simulink model "L4_SIM"  (R2018a)
settings: Solver=ode1  StartTime=0.0  StopTime=60  FixedStep=GLB_FIXED_STEP_SIZE_CPV  RelTol=1e-3  EnableMultiTasking=on
undefined symbols (not defined in the file or in its folder): Cf, Chassis, Cr, CYCLE_ACC1_2A__AdaptiveCruiseCtrlMode, CYCLE_ACC1_2A__AdaptiveCruiseCtrlSetSpeed, CYCLE_CCVS1_00__CruiseCtrlSetSpeed, CYCLE_CCVS1_00__WheelBasedVehicleSpeed, CYCLE_EEC1_00__EngSpeed, CYCLE_ETC1_00__TransDrivelineEngaged, CYCLE_ETC2_00__TransActualGearRatio, CYCLE_ETC7_03__TransMode1Indicator, CYCLE_GPS_Latitude, CYCLE_GPS_Longitude, CYCLE_LFE1_00__EngFuelRate, CYCLE_Net_Engine_Percent_Torque, CYCLE_SSI2_03__PitchAngleExRange, CYCLE_TIME, CYCLE_UTM_Origin_X, CYCLE_UTM_Origin_Y, CYCLE_Vehicle_Distance, DiscIntNeverNeededParam, ENUM_J1939_PCC_STATE_T, ENUM_J1939_SWITCH_T, ENUM_STEERING_WHEEL_ANGLE_SENSOR_TYPE_T, GLB_FIXED_STEP_SIZE_CPV, GLB_TRANS_LOSS_TRQ_GEAR_STEP_MPV, GLB_TRANS_LOSS_TRQ_SPD_STEP_MPV, GLB_TRANS_LOSS_TRQ_TABLE_DATA_MPV, GLB_TRANS_LOSS_TRQ_TRQ_STEP_MPV, GLB_VEHICLE_CONFIG_ACCEL_PED_GATEWAY_APV, heading_0, Iz, L4_Controller, lf, lr, position_0, ptc_matlab_lib, STEERCTRL_10ms, SUB_ECU_L4_MABX, SUB_L4_Task_10ms, SUB_L4_Task_10ms_SUB_STEERCTRL, SUB_PLANT_Chassis, Task_10ms, Vx_0
libraries: EmE_MBD_Blockset x81, PTC_MBDS_LIB x71, simulink x38, simulink_extras x1, SUB_L4_Task_10000ms x1, SUB_L4_Task_1000ms x1, SUB_L4_Task_100ms x1, SUB_L4_Task_10ms_SUB_APTC x1, SUB_L4_Task_10ms_SUB_BRKPEDARB x1, SUB_L4_Task_10ms_SUB_FAULT_MANAGER x1, SUB_L4_Task_10ms_SUB_STATE_CONTROL x1, simulink_need_slupdate x1
(part 6 of 6)

== system L4_SIM/Controllers/Virtual_Controllers/L4_MABX/L4_Controller/Task_10ms/Vehicle_speed_target/Determine_sigmoid_vehicle_speed_profile/Select_vehicle_speed_target_value ==
  Vehicle_speed_initial : Inport
  F_Enable : Inport  Port=2
  Distance_m : Inport  Port=3
  Vehicle_speed : Inport  Port=4
  Vehicle_speed_target : Inport  Port=5
  Position_vector_m : Inport  Port=6
  Vehicle_speed_vector_kph : Inport  Port=7
  MIN_VSPD_SIGMOID_INITIAL_KPH_APV : Inport  Port=8
  MIN_VSPD_SIGMOID_FINAL_KPH_APV : Inport  Port=9
  CPV1 : EmE_MBD_Blockset/Sources/CPV  conval=0.1
      settings: SourceProductName=PACCAR EmE MBD Blockset
  Gain1 : Gain  Gain=1/3.6
  If_Then_Else : EmE_MBD_Blockset/Signal Routing/If_Then_Else
      settings: SourceProductName=PACCAR EmE MBD Blockset
  Integrators : Subsystem
  Logical Operator : EmE_MBD_Blockset/Logic and Bit Operations/Logical Operator  Operator=OR  Inputs=2
      settings: SourceProductName=PACCAR EmE MBD Blockset
  Logical Operator2 : EmE_MBD_Blockset/Logic and Bit Operations/Logical Operator  Operator=AND  Inputs=2
      settings: SourceProductName=PACCAR EmE MBD Blockset
  Lookup Table Dynamic : simulink/Lookup Tables/Lookup Table Dynamic  LookUpMeth=Interpolation-Use End Values  OutDataType=fixdt('double')  OutScaling=[]  OutputDataTypeScalingMode=Specify via dialog  OutDataTypeStr=double  DoSatur=off
      settings: SourceProductName=Simulink
  Relational Operator : EmE_MBD_Blockset/Logic and Bit Operations/Relational Operator  func===
      settings: SourceProductName=PACCAR EmE MBD Blockset
  Relational Operator1 : EmE_MBD_Blockset/Logic and Bit Operations/Relational Operator  func=<
      settings: SourceProductName=PACCAR EmE MBD Blockset
  Relational Operator2 : EmE_MBD_Blockset/Logic and Bit Operations/Relational Operator  func=<
      settings: SourceProductName=PACCAR EmE MBD Blockset
  Relational Operator3 : EmE_MBD_Blockset/Logic and Bit Operations/Relational Operator  func=<
      settings: SourceProductName=PACCAR EmE MBD Blockset
  Terminator : Terminator
  Vehicle_speed_profile_sigmoid : Outport
  wires:
  Logical Operator2/1 -> Integrators/3(F_SetMax)  "F_set_max_distance_accumulated"
  CPV1/1 -> Relational Operator3/2
  Relational Operator1/1 -> Logical Operator/2
  Logical Operator/1 -> Logical Operator2/1
  Relational Operator3/1 -> Logical Operator/1
  Relational Operator/1 -> If_Then_Else/1
  Gain1/1 -> Integrators/2(Vehicle_speed_ms)
  Integrators/2(Distance_accumulated_m) -> Relational Operator/1, Lookup Table Dynamic/1
  MIN_VSPD_SIGMOID_FINAL_KPH_APV/1 -> Relational Operator2/2
  MIN_VSPD_SIGMOID_INITIAL_KPH_APV/1 -> Relational Operator1/2
  Relational Operator2/1 -> Logical Operator2/2
  Vehicle_speed_initial/1 -> Relational Operator1/1
  F_Enable/1 -> Integrators/1(F_Reset)
  Lookup Table Dynamic/1 -> If_Then_Else/3
  Vehicle_speed_vector_kph/1 -> Lookup Table Dynamic/3
  Integrators/1(Elasped_time_secs) -> Terminator/1
  Position_vector_m/1 -> Lookup Table Dynamic/2
  Vehicle_speed/1 -> Gain1/1, Relational Operator3/1
  Distance_m/1 -> Integrators/4(Max), Relational Operator/2
  If_Then_Else/1 -> Vehicle_speed_profile_sigmoid/1  "Vehicle_speed_profile_sigmoid"
  Vehicle_speed_target/1 -> Relational Operator2/1, If_Then_Else/2

== system L4_SIM/Plant/PlantModel/Chassis/Chassis_SL/Chassis/Vehicle Dynamics/Aero/Signed square ==
  In1 : Inport
  Math Function : Math  Operator=square  SaturateOnIntegerOverflow=on
  Product : Product  RndMeth=Zero
  Sign : Signum  ZeroCross=off
  Out1 : Outport
  wires:
  Product/1 -> Out1/1
  Sign/1 -> Product/2
  Math Function/1 -> Product/1
  In1/1 -> Sign/1, Math Function/1

== system L4_SIM/Controllers/Virtual_Controllers/L4_MABX/L4_Controller/Task_10ms/STEERCTRL_10ms/PID/PID/PID ==
  Init : Inport
  Reset_Integral : Inport  Port=2
  Err : Inport  Port=3
  K : Inport  Port=4
  Ti : Inport  Port=5
  Td : Inport  Port=6
  Ts : Inport  Port=7
  Sat_state : Inport  Port=8
  Add : Sum
  Add1 : Sum  Inputs=+++
  Add3 : Sum  Inputs=+-
  AntiWindup : Subsystem
  Divide : Product  Inputs=*/
  Divide1 : Product  Inputs=**/
  Product : Product  RndMeth=Zero
  Product1 : Product  RndMeth=Zero
  Switch : Switch  Criteria=u2 ~= 0
  Unit Delay : UnitDelay  SampleTime=-1
  Unit Delay1 : UnitDelay  SampleTime=-1
  Out1 : Outport
  P_Out : Outport  Port=2
  I_Out : Outport  Port=3
  D_Out1 : Outport  Port=4
  wires:
  Add3/1 -> D_Out1/1, Add1/3
  Unit Delay1/1 -> Add3/2
  Divide1/1 -> Unit Delay1/1, Add3/1
  [KpError] -> Divide1/2
  Td/1 -> Divide1/1
  Add1/1 -> Out1/1
  Add/1 -> I_Out/1, Add1/2, Switch/3
  Switch/1 -> Unit Delay/1
  Unit Delay/1 -> Add/2
  Divide/1 -> Product1/2
  Ti/1 -> Divide/2
  Ts/1 -> Divide/1, Divide1/3
  Product/1 -> [KpError], P_Out/1, Add1/1, Product1/1
  K/1 -> Product/2
  Err/1 -> Product/1
  Init/1 -> Switch/1
  Reset_Integral/1 -> Switch/2
  AntiWindup/1(I_update_clp) -> Add/1
  Product1/1 -> AntiWindup/1(I_update)
  Sat_state/1 -> AntiWindup/2(Sat_state)

== system L4_SIM/Controllers/Virtual_Controllers/L4_MABX/L4_Controller/Task_10ms/Vehicle_speed_target/Determine_sigmoid_vehicle_speed_profile/Determine_inhibit_sigmoid_vehicle_speed_profile/Capture_initial_vehicle_speed_value ==
  Vehicle_speed : Inport
  F_Enable : Inport  Port=2
  If_Then_Else : EmE_MBD_Blockset/Signal Routing/If_Then_Else
      settings: SourceProductName=PACCAR EmE MBD Blockset
  Unit_Delay : UnitDelay  SampleTime=-1
      settings: AttributesFormatString=IC: %<vinit>
  Vehicle_speed_initial : Outport
  wires:
  Vehicle_speed/1 -> If_Then_Else/2
  Unit_Delay/1 -> If_Then_Else/3
  F_Enable/1 -> If_Then_Else/1
  If_Then_Else/1 -> Vehicle_speed_initial/1, Unit_Delay/1  "Vehicle_speed_initial"

== system L4_SIM/Controllers/Virtual_Controllers/L4_MABX/L4_Controller/Task_10ms/Vehicle_speed_target/Determine_sigmoid_vehicle_speed_profile/Select_vehicle_speed_target_value/Integrators ==
  F_Reset : Inport
  Vehicle_speed_ms : Inport  Port=2
  F_SetMax : Inport  Port=3
  Max : Inport  Port=4
  CPV : EmE_MBD_Blockset/Sources/CPV  conval=1
      settings: SourceProductName=PACCAR EmE MBD Blockset
  CPV1 : EmE_MBD_Blockset/Sources/CPV  conval=1
      settings: SourceProductName=PACCAR EmE MBD Blockset
  CPV2 : EmE_MBD_Blockset/Sources/CPV  conval=1
      settings: SourceProductName=PACCAR EmE MBD Blockset
  CalculateDistance : Subsystem
  Discrete-Time Integrator : EmE_MBD_Blockset/Discrete/Discrete-Time Integrator  integrator_method_sel=Backward Euler
      settings: AttributesFormatString=%<integrator_method_sel>  SourceProductName=PACCAR EmE MBD Blockset
  dT : EmE_MBD_Blockset/Sources/dT
      settings: SourceProductName=PACCAR EmE MBD Blockset
  dT1 : EmE_MBD_Blockset/Sources/dT
      settings: SourceProductName=PACCAR EmE MBD Blockset
  Elasped_time_secs : Outport
  Distance_accumulated_m : Outport  Port=2
  wires:
  F_SetMax/1 -> CalculateDistance/5(F_SetMax)
  Max/1 -> CalculateDistance/6(Max)
  CPV2/1 -> Discrete-Time Integrator/2
  CPV1/1 -> CalculateDistance/3(K)
  dT1/1 -> CalculateDistance/4(dT)
  Discrete-Time Integrator/1 -> Elasped_time_secs/1  "Elasped_time_secs"
  F_Reset/1 -> Discrete-Time Integrator/1, CalculateDistance/1(F_Reset)
  Vehicle_speed_ms/1 -> CalculateDistance/2(U)
  CPV/1 -> Discrete-Time Integrator/3
  CalculateDistance/1(Y) -> Distance_accumulated_m/1  "Distance_accumulated_m"
  dT/1 -> Discrete-Time Integrator/4

== system L4_SIM/Controllers/Virtual_Controllers/L4_MABX/L4_Controller/Task_10ms/STEERCTRL_10ms/PID/PID/PID/AntiWindup ==
  I_update : Inport
  Sat_state : Inport  Port=2
  Constant : Constant  Value=0
  Constant1 : Constant
  Constant2 : Constant  Value=-1
  Constant3 : Constant
  Constant4 : Constant  Value=-1
  Constant5 : Constant  Value=2
  Logical Operator : Logic  Operator=OR  AllPortsSameDT=off  OutDataTypeStr=boolean
  Logical Operator1 : Logic  AllPortsSameDT=off  OutDataTypeStr=boolean
  Logical Operator2 : Logic  AllPortsSameDT=off  OutDataTypeStr=boolean
  Logical Operator3 : Logic  AllPortsSameDT=off  OutDataTypeStr=boolean
  Relational Operator1 : RelationalOperator  Operator=~=  OutDataTypeStr=boolean  RndMeth=Nearest
  Relational Operator2 : RelationalOperator  Operator=~=  OutDataTypeStr=boolean  RndMeth=Nearest
  Relational Operator3 : RelationalOperator  Operator===  OutDataTypeStr=boolean  RndMeth=Nearest
  Relational Operator4 : RelationalOperator  Operator===  OutDataTypeStr=boolean  RndMeth=Nearest
  Relational Operator5 : RelationalOperator  Operator=~=  OutDataTypeStr=boolean  RndMeth=Nearest
  Sign1 : Signum
  Switch1 : Switch  Criteria=u2 ~= 0
  I_update_clp : Outport
  wires:
  Switch1/1 -> I_update_clp/1
  I_update/1 -> Sign1/1, Switch1/1
  Constant1/1 -> Relational Operator1/2
  Sat_state/1 -> Relational Operator1/1, Relational Operator2/1, [Sat_state]
  Constant2/1 -> Relational Operator2/2
  Sign1/1 -> Relational Operator4/2, Relational Operator3/2
  Constant3/1 -> Relational Operator3/1
  Constant4/1 -> Relational Operator4/1
  Relational Operator2/1 -> Logical Operator1/2
  Relational Operator4/1 -> Logical Operator1/1
  Relational Operator3/1 -> Logical Operator2/2
  Relational Operator1/1 -> Logical Operator2/1
  Logical Operator1/1 -> Logical Operator/1
  Logical Operator2/1 -> Logical Operator/2
  Constant/1 -> Switch1/3
  Logical Operator3/1 -> Switch1/2
  Logical Operator/1 -> Logical Operator3/2
  Constant5/1 -> Relational Operator5/2
  [Sat_state] -> Relational Operator5/1
  Relational Operator5/1 -> Logical Operator3/1

== system L4_SIM/Controllers/Virtual_Controllers/L4_MABX/L4_Controller/Task_10ms/Vehicle_speed_target/Determine_sigmoid_vehicle_speed_profile/Select_vehicle_speed_target_value/Integrators/CalculateDistance ==
  F_Reset : Inport
  U : Inport  Port=2
  K : Inport  Port=3
  dT : Inport  Port=4
  F_SetMax : Inport  Port=5
  Max : Inport  Port=6
  Add : Sum  InputSameDT=on
  CPV : EmE_MBD_Blockset/Sources/CPV  conval=0
      settings: SourceProductName=PACCAR EmE MBD Blockset
  If_Then_Else : EmE_MBD_Blockset/Signal Routing/If_Then_Else
      settings: SourceProductName=PACCAR EmE MBD Blockset
  MinMax : MinMax  Inputs=2  InputSameDT=on
  Product1 : Product  Inputs=3  InputSameDT=on
  Unit Delay Resettable External IC1 : simulink_need_slupdate/Unit Delay Resettable External IC  tsamp=-1
      settings: SourceProductName=Simulink  SourceProductBaseCode=SL
  Y : Outport  OutputWhenDisabled=reset  InitialOutput=0
  wires:
  F_Reset/1 -> Unit Delay Resettable External IC1/2
  Product1/1 -> Add/2
  Add/1 -> MinMax/2
  CPV/1 -> Unit Delay Resettable External IC1/3
  Unit Delay Resettable External IC1/1 -> Add/1
  If_Then_Else/1 -> Y/1, Unit Delay Resettable External IC1/1
  MinMax/1 -> If_Then_Else/3
  F_SetMax/1 -> If_Then_Else/1
  Max/1 -> If_Then_Else/2, MinMax/1
  dT/1 -> Product1/3
  K/1 -> Product1/1
  U/1 -> Product1/2

== stateflow chart L4_SIM/Controllers/Virtual_Controllers/L4_MABX/L4_Controller/Task_10ms/Vehicle_speed_target/Determine_sigmoid_vehicle_speed_profile/VehicleSpeedSetpointDynamicCalculation ==
  state CalculateAcceleration34 [function]
    (default) -> (junction 180) : {num = 2 * (AccelerationInitialLimited *  AccelerationFinalLimited ...
        |     - AccelerationInitialLimited * Jerk56 * TimeFinal ...
        |     + Jerk56 * (VelocityFinalLimited - VelocityInitialLimited)) ...
        |     - AccelerationInitialLimited^2 - AccelerationFinalLimited^2;
        |
        | den = 2 * ((VelocityFinalLimited - VelocityInitialLimited) ...
        |     - AccelerationFinalLimited * TimeFinal) ...
        |     + Jerk56 * TimeFinal^2;
        |
        | Jerk12 = sign(Jerk12) * max(abs(Jerk12), abs(num / den) + 0.001);
        | Jerk12 = max(-10,min(10,Jerk12));
        |
        | Calculate_abc}
    (junction 180) -> (junction 181) [order 1] : [abs(a) < 0.01 ]
    (junction 180) -> (junction 205) [order 2]
    (junction 181) -> (junction 183) : {Jerk12 = Jerk56;
        | Calculate_abc
        | Acceleration34 = - c / b;
        | AlternateMethod = false;}
    (junction 205) -> (junction 291) [order 1] : [b^2 <= 4 * a * c]
    (junction 205) -> (junction 288) [order 2] : {Acceleration34 = (- b + (b^2 - 4 * a * c)^0.5) / (2 * a);
        | AlternateMethod = false;}
    (junction 291) -> (junction 290) : {CalculateAlternate_abc
        | Acceleration34 = - b / (2 * a);
        | AlternateMethod = true;}
    (junction 290) -> (junction 288)
    (junction 183) -> (junction 290)
    (junction 288) -> (junction 189)
  state Calculate_abc [function]
    (default) -> (junction 164) : {a = Jerk56 - Jerk12;
        | b = 2 * (AccelerationFinalLimited * Jerk12 - AccelerationInitialLimited * Jerk56 - Jerk12 * Jerk56 * TimeFinal);
        | c = 2 * Jerk12 * Jerk56 * (VelocityFinalLimited - VelocityInitialLimited) + Jerk56 * AccelerationInitialLimited^2 - Jerk12 * AccelerationFinalLimited^2;}
  state CalculateAlternate_abc [function]
    (default) -> (junction 287) : {a = 1;
        | b = 2 * (Jerk56 * (TimeFinal - 0.005) - AccelerationFinalLimited);
        | c = 2 * Jerk56 * (VelocityInitialLimited - VelocityFinalLimited) + AccelerationFinalLimited^2;}
  (default) -> (junction 85)
  (junction 85) -> (junction 86) [order 1] : [Enable]
  (junction 85) -> (junction 87) [order 2]
  (junction 86) -> (junction 236) : {PositionFinalLimited = max(0.001,PositionFinal);  % limit minimum distance so that values in PositionVectorRaw are in increasing order
      |
      | VelocityInitialLimited = max(0.1,VelocityInitial);  % limit to make sure FinalTime calculation does not divide by zero
      | VelocityFinalLimited = max(0.1,VelocityFinal);  % limit to make sure FinalTime calculation does not divide by zero
      |
      | TimeFinal = 2 * PositionFinalLimited / (VelocityInitialLimited + VelocityFinalLimited);  % first approximation for total time
      | TimeFinal = max(0.007, TimeFinal);  % limit to make sure values in JerkVectorRaw are in increasing order and divide by zero protection
      |  AccelerationAverage = (VelocityFinalLimited - VelocityInitialLimited) / TimeFinal;   % acceleration with straight line velocity change
      | TimeFinal = 2 * TimeFinal;  % increase initial estimate two times to make sure solution is within search range
      | }
  (junction 236) -> (junction 237) [order 1] : [VelocityFinalLimited > VelocityInitialLimited]
  (junction 236) -> (junction 38) [order 2] : {% deceleration sigmoid limits
      | AccelerationInitialLimited = max(AccelerationAverage, min(0, AccelerationInitial));
      | AccelerationFinalLimited = max(AccelerationAverage, min(0, AccelerationFinal));}
  (junction 237) -> (junction 239) : {% acceleration sigmoid limits
      | AccelerationInitialLimited = max(0, min(AccelerationAverage, AccelerationInitial));
      | AccelerationFinalLimited = max(0, min(AccelerationAverage, AccelerationFinal));}
  (junction 239) -> (junction 38)
  (junction 38) -> (junction 21) : {DeltaTimeFinal = TimeFinal;  % initialize DeltaTimeFinal term for binary search
      | i = 1;}
  (junction 21) -> (junction 19) [order 1] : % TimeFinal
      | % Binary Search
      |
      | [i <= 15]
  (junction 19) -> (junction 115) : {JerkFinalMinimum = 2 * (VelocityInitialLimited - VelocityFinalLimited + AccelerationFinalLimited * TimeFinal) / TimeFinal^2;}
  (junction 115) -> (junction 117) [order 1] : [VelocityFinalLimited > VelocityInitialLimited]
  (junction 115) -> (junction 269) [order 2] : {% deceleration
      | Jerk12 = -JerkMagnitudeInitial;
      | Jerk56 = max(abs(JerkFinalMinimum), JerkMagnitudeFinal);}
  (junction 117) -> (junction 119) : {% acceleration
      | Jerk12 = JerkMagnitudeInitial;
      | Jerk56 = -max(abs(JerkFinalMinimum), JerkMagnitudeFinal);}
  (junction 119) -> (junction 269)
  (junction 269) -> (junction 25) : {CalculateAcceleration34}
  (junction 25) -> (junction 143) [order 1] : [abs(Acceleration34 - AccelerationAverage) < 0.001]
  (junction 25) -> (junction 297) [order 2]
  (junction 143) -> (junction 149) : {Time12 = 0.002;
      | Time56 = 0.002;
      |
      | TimeVectorRaw = [0; Time12 - 0.001; Time12 + 0.001; ...
      |     TimeFinal - Time56 - 0.001; TimeFinal - Time56 + 0.001;TimeFinal];
      |
      | JerkVectorRaw = [0; 0; 0; 0; 0; 0];
      | AccelerationVectorRaw(1) = AccelerationAverage;}
  (junction 297) -> (junction 299) [order 1] : [AlternateMethod]
  (junction 297) -> (junction 156) [order 2] : {Time12 = max(0.002, (Acceleration34 - AccelerationInitialLimited) / Jerk12);
      | Time56 = max(0.002, (AccelerationFinalLimited - Acceleration34) / Jerk56);
      |
      | TimeVectorRaw = [0; Time12 - 0.001; Time12 + 0.001; ...
      |     TimeFinal - Time56 - 0.001; TimeFinal - Time56 + 0.001;TimeFinal];
      |
      | JerkVectorRaw = [Jerk12; Jerk12; 0; 0; Jerk56; Jerk56];
      | AccelerationVectorRaw(1) = AccelerationInitialLimited;}
  (junction 299) -> (junction 301) : {Time12 = 0.002;
      | Time56 = max(0.002, (AccelerationFinalLimited - Acceleration34) / Jerk56);
      |
      | TimeVectorRaw = [0; Time12 - 0.001; Time12 + 0.001; ...
      |     TimeFinal - Time56 - 0.001; TimeFinal - Time56 + 0.001;TimeFinal];
      |
      | JerkVectorRaw = [0; 0; 0; 0; Jerk56; Jerk56];
      | AccelerationVectorRaw(1) = Acceleration34;}
  (junction 301) -> (junction 156)
  (junction 149) -> (junction 301)
  (junction 22) -> (junction 21) : {i = i + 1;}
  (junction 21) -> (junction 23) [order 2]
  (junction 156) -> (junction 32) : {VelocityVectorRaw(1) = VelocityInitialLimited;
      | PositionVectorRaw(1) = 0;
      | j = 2;}
  (junction 32) -> (junction 35) [order 1] : [j <= 6]
  (junction 35) -> (junction 31) : {DeltaTime = TimeVectorRaw(j) - TimeVectorRaw(j-1);
      | AverageJerk = 0.5 * (JerkVectorRaw(j-1) + JerkVectorRaw(j));
      | AccelerationVectorRaw(j) = AccelerationVectorRaw(j-1) + JerkVectorRaw(j-1) * DeltaTime;
      | VelocityVectorRaw(j) = VelocityVectorRaw(j-1) + AccelerationVectorRaw(j-1) * DeltaTime + 0.5 * JerkVectorRaw(j-1) * DeltaTime^2;
      | PositionVectorRaw(j) = PositionVectorRaw(j-1) + VelocityVectorRaw(j-1) * DeltaTime + 0.5 * AccelerationVectorRaw(j-1) * DeltaTime^2 + (JerkVectorRaw(j-1) / 6) * DeltaTime^3;}
  (junction 31) -> (junction 32) : {j = j + 1;}
  (junction 32) -> (junction 56) [order 2] : {PositionError = PositionVectorRaw(end) - PositionFinalLimited;
      | DeltaTimeFinal = 0.5 * DeltaTimeFinal;  % reduce DeltaTimeFinal by 50 percent on each iteration of the search
      | }
  (junction 56) -> (junction 57) [order 1] : [(PositionError < 0) && (VelocityVectorRaw(end) > 0)]
  (junction 56) -> (junction 59) [order 2] : {TimeFinal = TimeFinal - DeltaTimeFinal;}
  (junction 57) -> (junction 58) : {TimeFinal = TimeFinal + DeltaTimeFinal;}
  (junction 58) -> (junction 59)
  (junction 59) -> (junction 22) : {TimeFinal = max(0.007, TimeFinal);}
  (junction 23) -> (junction 87)
  (junction 87) -> (junction 92)
  data: TimeVectorRaw output size=6 =[0:0.001:0.005]'; PositionVectorRaw output size=6 =[0:0.001:0.005]'; VelocityVectorRaw output size=6 =zeros(6,1); AccelerationVectorRaw output size=6 =zeros(6,1); JerkVectorRaw output size=6 =zeros(6,1); Enable input boolean; PositionFinal input; VelocityInitial input; VelocityFinal input; AccelerationInitial input; AccelerationFinal input; TimeFinal local double; AccelerationAverage local double; DeltaTimeFinal local double; i local uint8; j local uint8; DeltaTime local double; AverageJerk local double; PositionError local double; JerkError local double; PositionFinalLimited local double; VelocityInitialLimited local double; VelocityFinalLimited local double; AccelerationInitialLimited local double; AccelerationFinalLimited local double; Jerk56 local double; Jerk12 local double; JerkMagnitudeInitial input; JerkMagnitudeFinal input; a local double; b local double; c local double; Acceleration34 local double; Time12 local double; Time56 local double; JerkFinalMinimum local double; AlternateMethod local boolean; num local double; den local double

== stateflow chart L4_SIM/Controllers/Virtual_Controllers/L4_MABX/L4_Controller/Task_10ms/Vehicle_speed_target/Determine_sigmoid_vehicle_speed_profile/TwentyPointVectorCalculation ==
  (default) -> (junction 85)
  (junction 85) -> (junction 86) [order 1] : [Enable]
  (junction 85) -> (junction 87) [order 2]
  (junction 86) -> (junction 21) : {TimeVector(1) = TimeVectorRaw(1);
      | JerkVector(1) = JerkVectorRaw(1);
      | AccelerationVector(1) = AccelerationVectorRaw(1);
      | VelocityVector(1) = VelocityVectorRaw(1);
      | PositionVector(1) = PositionVectorRaw(1);
      |
      | TimeIncrement = (TimeVectorRaw(2) - TimeVectorRaw(1)) / 10;
      | i = 2;}
  (junction 21) -> (junction 19) [order 1] : [i <= 10]
  (junction 19) -> (junction 22) : {TimeVector(i) = TimeVector(i-1) + TimeIncrement;
      | DeltaTime = TimeVector(i) - TimeVectorRaw(1);
      | JerkVector(i) = JerkVectorRaw(1);
      | AccelerationVector(i) = AccelerationVectorRaw(1) + JerkVectorRaw(1) * DeltaTime;
      | VelocityVector(i) = VelocityVectorRaw(1) + AccelerationVectorRaw(1) * DeltaTime + 0.5 * JerkVectorRaw(1) * DeltaTime^2;
      | PositionVector(i) = PositionVectorRaw(1) + VelocityVectorRaw(1) * DeltaTime + 0.5 * AccelerationVectorRaw(1) * DeltaTime^2 + (JerkVectorRaw(1) / 6) * DeltaTime^3;
      | PositionVector(i) = max(PositionVector(i-1) + 0.0001, PositionVector(i));}
  (junction 22) -> (junction 21) : {i = i + 1;}
  (junction 21) -> (junction 129) [order 2] : {TimeVector(11) = TimeVectorRaw(2);
      | JerkVector(11) = JerkVectorRaw(2);
      | AccelerationVector(11) = AccelerationVectorRaw(2);
      | VelocityVector(11) = VelocityVectorRaw(2);
      | PositionVector(11) = max(PositionVector(10) + 0.0001, PositionVectorRaw(2));
      |
      | TimeVector(12) = TimeVectorRaw(3);
      | JerkVector(12) = JerkVectorRaw(3);
      | AccelerationVector(12) = AccelerationVectorRaw(3);
      | VelocityVector(12) = VelocityVectorRaw(3);
      | PositionVector(12) = max(PositionVector(11) + 0.0001, PositionVectorRaw(3));
      |
      | TimeIncrement = (TimeVectorRaw(4) - TimeVectorRaw(3)) / 10;
      | i = 13;}
  (junction 129) -> (junction 128) [order 1] : [i <= 21]
  (junction 128) -> (junction 130) : {TimeVector(i) = TimeVector(i-1) + TimeIncrement;
      | DeltaTime = TimeVector(i) - TimeVectorRaw(3);
      | JerkVector(i) = JerkVectorRaw(3);
      | AccelerationVector(i) = AccelerationVectorRaw(3) + JerkVectorRaw(3) * DeltaTime;
      | VelocityVector(i) = VelocityVectorRaw(3) + AccelerationVectorRaw(3) * DeltaTime + 0.5 * JerkVectorRaw(3) * DeltaTime^2;
      | PositionVector(i) = PositionVectorRaw(3) + VelocityVectorRaw(3) * DeltaTime + 0.5 * AccelerationVectorRaw(3) * DeltaTime^2 + (JerkVectorRaw(3) / 6) * DeltaTime^3;
      | PositionVector(i) = max(PositionVector(i-1) + 0.0001, PositionVector(i));}
  (junction 130) -> (junction 129) : {i = i + 1;}
  (junction 129) -> (junction 109) [order 2] : {TimeVector(22) = TimeVectorRaw(4);
      | JerkVector(22) = JerkVectorRaw(4);
      | AccelerationVector(22) = AccelerationVectorRaw(4);
      | VelocityVector(22) = VelocityVectorRaw(4);
      | PositionVector(22) = max(PositionVector(21) + 0.0001, PositionVectorRaw(4));
      |
      | TimeVector(23) = TimeVectorRaw(5);
      | JerkVector(23) = JerkVectorRaw(5);
      | AccelerationVector(23) = AccelerationVectorRaw(5);
      | VelocityVector(23) = VelocityVectorRaw(5);
      | PositionVector(23) = max(PositionVector(22) + 0.0001, PositionVectorRaw(5));
      |
      | TimeIncrement = (TimeVectorRaw(6) - TimeVectorRaw(5)) / 10;
      | i = 24;}
  (junction 109) -> (junction 107) [order 1] : [i <= 32]
  (junction 107) -> (junction 108) : {TimeVector(i) = TimeVector(i-1) + TimeIncrement;
      | DeltaTime = TimeVector(i) - TimeVectorRaw(5);
      | JerkVector(i) = JerkVectorRaw(5);
      | AccelerationVector(i) = AccelerationVectorRaw(5) + JerkVectorRaw(5) * DeltaTime;
      | VelocityVector(i) = VelocityVectorRaw(5) + AccelerationVectorRaw(5) * DeltaTime + 0.5 * JerkVectorRaw(5) * DeltaTime^2;
      | PositionVector(i) = PositionVectorRaw(5) + VelocityVectorRaw(5) * DeltaTime + 0.5 * AccelerationVectorRaw(5) * DeltaTime^2 + (JerkVectorRaw(5) / 6) * DeltaTime^3;
      | PositionVector(i) = max(PositionVector(i-1) + 0.0001, PositionVector(i));}
  (junction 108) -> (junction 109) : {i = i + 1;}
  (junction 109) -> (junction 23) [order 2] : {TimeVector(33) = TimeVectorRaw(6);
      | JerkVector(33) = JerkVectorRaw(6);
      | AccelerationVector(33) = AccelerationVectorRaw(6);
      | VelocityVector(33) = VelocityVectorRaw(6);
      | PositionVector(33) = max(PositionVector(32) + 0.0001, PositionVectorRaw(6));}
  (junction 23) -> (junction 87)
  (junction 87) -> (junction 92)
  data: TimeVector output size=33 =[0:0.001:0.032]'; PositionVector output size=33 =[0:0.001:0.032]'; VelocityVector output size=33 =zeros(33,1); AccelerationVector output size=33 =zeros(33,1); JerkVector output size=33 =zeros(33,1); Enable input; PositionFinal input; TimeVectorRaw input; PositionVectorRaw input; VelocityVectorRaw input; AccelerationVectorRaw input; JerkVectorRaw input; i local uint8; DeltaTime local double; TimeIncrement local double

== matlab function L4_SIM/Plant/PlantModel/Navigation/MATLAB Function1 ==
  data: Vx input; Vnav output; Vy input; heading input
function Vnav  = body2nav(Vx, Vy, heading)

Vnav = [0 0]';

Vnav(1) =  Vx*cos(heading) - Vy*sin(heading);
Vnav(2) =  Vx*sin(heading) + Vy*cos(heading);

== matlab function L4_SIM/Plant/PlantModel/Chassis/Chassis_SL/Chassis/Trailer Model/wrap to pi1 ==
  data: u input; y output
function y = fcn(u)
if (u>pi)
    y=u-2*pi;
elseif (u<-pi)
    y=u+2*pi;
else
    y=u;
end

== matlab function L4_SIM/Controllers/Drive_Cycle/DriveCycle/MATLAB Function ==
  data: x output; Lat input; y output; Lon input
function  [x,y] = deg2utm(Lat,Lon)
% -------------------------------------------------------------------------
% [x,y,utmzone] = deg2utm(Lat,Lon)
%
% Description: Function to convert lat/lon vectors into UTM coordinates (WGS84).
% Some code has been extracted from UTM.m function by Gabriel Ruiz Martinez.
%
% Inputs:
%    Lat: Latitude vector.   Degrees.  +ddd.ddddd  WGS84
%    Lon: Longitude vector.  Degrees.  +ddd.ddddd  WGS84
%
% Outputs:
%    x, y , utmzone.   See example
%
% Example 1:
%    Lat=[40.3154333; 46.283900; 37.577833; 28.645650; 38.855550; 25.061783];
%    Lon=[-3.4857166; 7.8012333; -119.95525; -17.759533; -94.7990166; 121.640266];
%    [x,y,utmzone] = deg2utm(Lat,Lon);
%    fprintf('%7.0f ',x)
%       458731  407653  239027  230253  343898  362850
%    fprintf('%7.0f ',y)
%      4462881 5126290 4163083 3171843 4302285 2772478
%    utmzone =
%       30 T
%       32 T
%       11 S
%       28 R
%       15 S
%       51 R
%
% Example 2: If you have Lat/Lon coordinates in Degrees, Minutes and Seconds
%    LatDMS=[40 18 55.56; 46 17 2.04];
%    LonDMS=[-3 29  8.58;  7 48 4.44];
%    Lat=dms2deg(mat2dms(LatDMS)); %convert into degrees
%    Lon=dms2deg(mat2dms(LonDMS)); %convert into degrees
%    [x,y,utmzone] = deg2utm(Lat,Lon)
%
% Author: 
%   Rafael Palacios
%   Universidad Pontificia Comillas
%   Madrid, Spain
% Version: Apr/06, Jun/06, Aug/06, Aug/06
% Aug/06: fixed a problem (found by Rodolphe Dewarrat) related to southern 
%    hemisphere coordinates. 
% Aug/06: corrected m-Lint warnings
%-------------------------------------------------------------------------

% Argument checking
%
narginchk(2, 2);  %2 arguments required
n1=length(Lat);
n2=length(Lon);
if (n1~=n2)
   error('Lat and Lon vectors should have the same length');
end


% Memory pre-allocation
%
x=zeros(n1,1);
y=zeros(n1,1);

% Main Loop
%
for i=1:n1
   la=Lat(i);
   lo=Lon(i);

   sa = 6378137.000000 ; sb = 6356752.314245;
         
   %e = ( ( ( sa ^ 2 ) - ( sb ^ 2 ) ) ^ 0.5 ) / sa;
   e2 = ( ( ( sa ^ 2 ) - ( sb ^ 2 ) ) ^ 0.5 ) / sb;
   e2cuadrada = e2 ^ 2;
   c = ( sa ^ 2 ) / sb;
   %alpha = ( sa - sb ) / sa;             %f
   %ablandamiento = 1 / alpha;   % 1/f

   lat = la * ( pi / 180 );
   lon = lo * ( pi / 180 );

   Huso = fix( ( lo / 6 ) + 31);
   S = ( ( Huso * 6 ) - 183 );
   deltaS = lon - ( S * ( pi / 180 ) );


   a = cos(lat) * sin(deltaS);
   epsilon = 0.5 * log( ( 1 +  a) / ( 1 - a ) );
   nu = atan( tan(lat) / cos(deltaS) ) - lat;
   v = ( c / ( ( 1 + ( e2cuadrada * ( cos(lat) ) ^ 2 ) ) ) ^ 0.5 ) * 0.9996;
   ta = ( e2cuadrada / 2 ) * epsilon ^ 2 * ( cos(lat) ) ^ 2;
   a1 = sin( 2 * lat );
   a2 = a1 * ( cos(lat) ) ^ 2;
   j2 = lat + ( a1 / 2 );
   j4 = ( ( 3 * j2 ) + a2 ) / 4;
   j6 = ( ( 5 * j4 ) + ( a2 * ( cos(lat) ) ^ 2) ) / 3;
   alfa = ( 3 / 4 ) * e2cuadrada;
   beta = ( 5 / 3 ) * alfa ^ 2;
   gama = ( 35 / 27 ) * alfa ^ 3;
   Bm = 0.9996 * c * ( lat - alfa * j2 + beta * j4 - gama * j6 );
   xx = epsilon * v * ( 1 + ( ta / 3 ) ) + 500000;
   yy = nu * v * ( 1 + ta ) + Bm;

   if (yy<0)
       yy=9999999+yy;
   end

   x(i)=xx;
   y(i)=yy;
   
end

== stateflow chart L4_SIM/Plant/PlantModel/Chassis/Chassis_SL/Transmission Simple ModeNo SDL/Main Clutch/Clutch ==
  state Init
    entry: State=1;
  state Open
    entry: State=2;
    entry: ClutchForce=0;
    during:TrqOutOut=0;
    during:TrqOutIn=0;
  state ReverseSlip
    en:State=4;
    during:ClutchForce = ClutchForce + k*GLB_FIXED_STEP_SIZE_CPV;
    during:TrqOutIn=-2/3*Radius*Friction*ClutchForce;
    during:TrqOutOut=TrqOutOut;
  state ForwardSlip
    en:State=3;
    during:ClutchForce = ClutchForce + k*GLB_FIXED_STEP_SIZE_CPV;
    during:TrqOutOut=2/3*Radius*Friction*ClutchForce;
    during:TrqOutIn=TrqOutOut;
  state Locked
    en:State=5;
    entry: ClutchForce=10000;
    during:TrqOutOut=TrqIn;
    during:TrqOutIn=0;
  (default) -> Init
  Init -> Open
  ReverseSlip -> Open [order 1] : [Act<0.5]
  Locked -> Open : [Act<0.5]
  ForwardSlip -> Open [order 2] : [Act<0.5]
  Open -> (junction 29) : [Act>=0.5]
  (junction 29) -> ReverseSlip [order 2] : [EngSpd<TransSpd]
  (junction 29) -> ForwardSlip [order 1] : [EngSpd>=TransSpd]
  ReverseSlip -> ForwardSlip [order 3] : [EngSpd>=TransSpd]
  ForwardSlip -> ReverseSlip [order 3] : [EngSpd<TransSpd]
  ReverseSlip -> Locked [order 2] : [abs(EngSpd-TransSpd)<SpdTol]
  ForwardSlip -> Locked [order 1] : [abs(EngSpd-TransSpd)<SpdTol]
  data: Act input; State output; TrqIn input; EngSpd input; TransSpd input; TrqOutOut output; k input; SpdTol input; TrqOutIn output; Radius input size=1; Friction input size=1; ClutchForce local; GLB_FIXED_STEP_SIZE_CPV parameter

== matlab function L4_SIM/Controllers/Operator/Subsystem/HeadingController/MATLAB Function ==
  data: heading output; xN input; yN input; target_waypoint input
function heading   = calc_target_waypoint(xN, yN, target_waypoint)
 
heading = atan2(target_waypoint(2)-yN,target_waypoint(1)-xN);
if heading < 0
    heading=heading+2*pi;

end

== matlab function L4_SIM/Controllers/Virtual_Controllers/L4_MABX/L4_Controller/Task_10ms/STEERCTRL_10ms/SteerController/Error Calc ==
  data: current input; target input; error output
function error = calc_error(current, target)

error = target - current;

if error < -pi
    error = error + 2*pi;
elseif error > pi
        error = error - 2*pi;
        
end

== stateflow chart L4_SIM/Controllers/Virtual_Controllers/L4_MABX/L4_Controller/Task_10ms/STEERCTRL_10ms/slew/Chart ==
  state init
    en:stateChange=uint8(0);
  state ZeroLanes
    en:stateChange=uint8(1);
  state OneLane
    en:stateChange=uint8(1);
  state ZeroLanes1
    en:stateChange=uint8(0);
  state OneLane1
    en:stateChange=uint8(0);
  state TwoLanes
    en:stateChange=uint8(1);
  state TwoLanes1
    en:stateChange=uint8(0);
  TwoLanes1 -> init : [numLanePoints<uint8(18)]
  (default) -> init
  init -> TwoLanes [order 2] : [numLanePoints>uint8(18)]
  OneLane1 -> init : [numLanePoints<uint8(3) ||numLanePoints>uint8(18)]
  init -> OneLane [order 3] : [numLanePoints>uint8(3)]
  ZeroLanes1 -> init : [numLanePoints>uint8(3)]
  init -> ZeroLanes [order 1] : [numLanePoints<=uint8(3)]
  ZeroLanes -> ZeroLanes1
  OneLane -> OneLane1
  TwoLanes -> TwoLanes1
  data: numLanePoints input uint8; stateChange output uint8
